simulink model "SimulinIntroExample"  (R2025b)
settings: Solver=VariableStepAuto  StartTime=0.0  StopTime=10.0  RelTol=1e-3
undefined symbols (not defined in the file or in its folder): brake_force_table, Desired_speed, K, speed_table
settings Model: Creator=ATuck  LastModifiedBy=ATuck

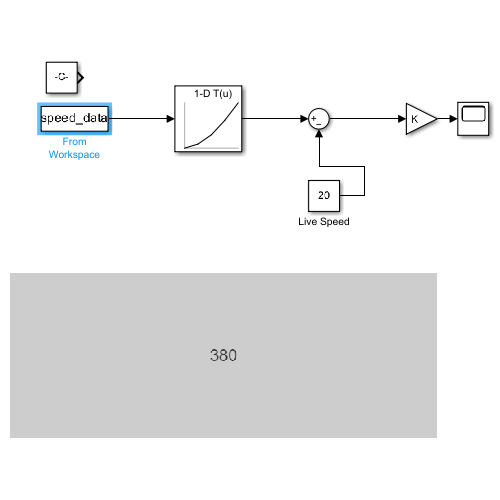
[thumbnail: Simulink's stored preview of the top-level diagram]
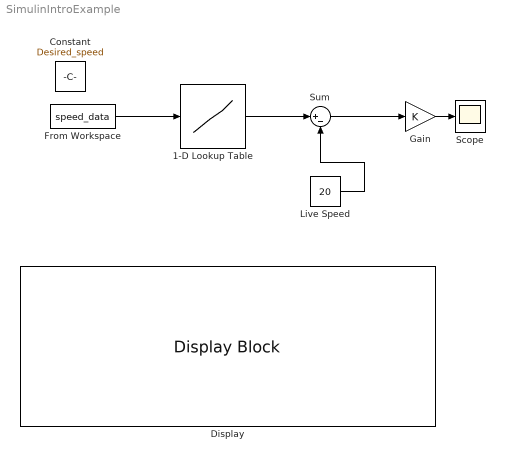
== system SimulinIntroExample ==
  1-D Lookup Table : Lookup_n-D  NumberOfTableDimensions=1  BreakpointsForDimension1=speed_table  Table=brake_force_table  InternalRulePriority=Speed  RndMeth=Simplest
  Constant : Constant  Value=Desired_speed
  Display : DisplayBlock  LabelPosition=Hide  Transparency=1  GridColor=[0.502, 0.502, 0.502]
  From Workspace : FromWorkspace  VariableName=speed_data  SampleTime=0.1
  Gain : Gain  Gain=K
  Live Speed : Constant  Value=20
  Scope : Scope
      settings: ActiveDisplayYMinimum=118.50000000000001  ActiveDisplayYMaximum=493.5
  Sum : Sum  Inputs=|+-
  wires:
  From Workspace/1 -> 1-D Lookup Table/1
  1-D Lookup Table/1 -> Sum/1
  Live Speed/1 -> Sum/2
  Sum/1 -> Gain/1
  Gain/1 -> Scope/1
